simulink model "lumlumLQR_simulink_model"  (R2020a)
settings: Solver=VariableStepAuto  StartTime=0.0  StopTime=10.0  RelTol=1e-3
values from neighbouring files (symbols this model uses):
  A_ = [0 1;0 -1/5]    [lumlumLQR.m]
  B_ = [0; 1]    [lumlumLQR.m]
  K_ = lqr(A_,B_,Q_,R_)    [lumlumLQR.m]
  x0 = [72*pi/180 ... (first row only)    [lumdownload.m]    (also in lumlumLQR.m = [pi;-2])
settings Model: Creator=Khojasteh Mirza  LastModifiedBy=Khojasteh Mirza

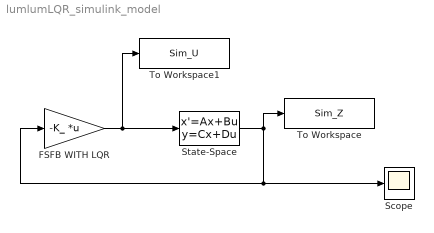
== system lumlumLQR_simulink_model ==
  FSFB WITH LQR : Gain  Gain=-K_  Multiplication=Matrix(K*u)
  Scope : Scope
  State-Space : StateSpace  A=A_  B=B_  C=eye(2)  D=zeros(2,1)  InitialCondition=x0
  To Workspace : ToWorkspace  VariableName=Sim_Z  SaveFormat=Structure With Time  SampleTime=-1
  To Workspace1 : ToWorkspace  VariableName=Sim_U  SaveFormat=Structure With Time  SampleTime=-1
  wires:
  FSFB WITH LQR/1 -> To Workspace1/1, State-Space/1
  State-Space/1 -> To Workspace/1, Scope/1, FSFB WITH LQR/1
